simulink model "surgicalControl"  (R2016b)
settings: Solver=FixedStepAuto  StartTime=0.0  StopTime=100.0  RelTol=1e-3
libraries: simulink x3
settings Model: Creator=daniel  LastModifiedBy=migf1

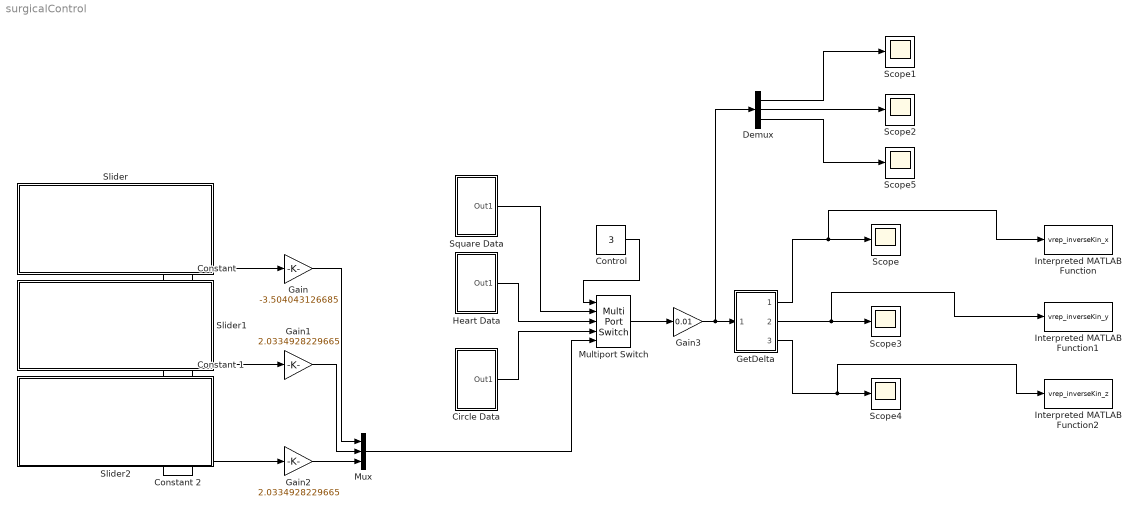
== system surgicalControl ==
  " GetDelta " : Subsystem
  " Constant " : Constant
  " Constant 1" : Constant
  " Constant 2" : Constant
  "Circle Data " : Subsystem
  "Control " : Constant  Value=3
  Demux : Demux  Outputs=3
  Gain : Gain  Gain=-3.504043126685
  Gain1 : Gain  Gain=2.0334928229665
  Gain2 : Gain  Gain=2.0334928229665
  Gain3 : Gain  Gain=0.01
  "Heart Data " : Subsystem
  Interpreted MATLAB Function : MATLABFcn  MATLABFcn=vrep_inverseKin_x
  Interpreted MATLAB Function1 : MATLABFcn  MATLABFcn=vrep_inverseKin_y
  Interpreted MATLAB Function2 : MATLABFcn  MATLABFcn=vrep_inverseKin_z
  Multiport Switch : MultiPortSwitch  Inputs=4
  Mux : Mux  Inputs=3
  Scope{,1..5} (6 alike) : Scope
  Slider : Subsystem  DialogController=hmiCreateDDGDialog  IsWebBlock=on  mask(MWDashboardBlock){webBlockId=4f94596f-dd6d-4e5e-bddc-7a8d913927f9, webBlockType=slider, ShowInLibBrowser=on, ShowInitialText=on, HMISrcModelName=surgicalControl}
      mask prompts: webBlockId "WebBlock Id"; webBlockType "WebBlock Type"; HMISrcModelName "Source Model"
      mask help: SimulinkHMI:dialogs:SliderDialogDesc
      mask Help: helpview([docroot '/mapfiles/simulink.map'], 'hmi_slider')
      mask Display:
      | if strcmp(get_param(bdroot(gcb),'BlockDiagramType'), 'library')
      |     image([(matlabroot) '/toolbox/simulink/hmi/icons/Slider.png']);
      | end
  Slider1 : Subsystem  DialogController=hmiCreateDDGDialog  IsWebBlock=on  mask(MWDashboardBlock){webBlockId=8aa996ad-7cd4-40fc-9a04-6a85939aea5d, webBlockType=slider, ShowInLibBrowser=on, ShowInitialText=on, HMISrcModelName=surgicalControl}
      mask prompts: webBlockId "WebBlock Id"; webBlockType "WebBlock Type"; HMISrcModelName "Source Model"
      mask help: SimulinkHMI:dialogs:SliderDialogDesc
      mask Help: helpview([docroot '/mapfiles/simulink.map'], 'hmi_slider')
      mask Display:
      | if strcmp(get_param(bdroot(gcb),'BlockDiagramType'), 'library')
      |     image([(matlabroot) '/toolbox/simulink/hmi/icons/Slider.png']);
      | end
  Slider2 : Subsystem  DialogController=hmiCreateDDGDialog  IsWebBlock=on  mask(MWDashboardBlock){webBlockId=1ddf6fd9-0225-4881-82ca-a25e179e2ab9, webBlockType=slider, ShowInLibBrowser=on, ShowInitialText=on, HMISrcModelName=surgicalControl}
      mask prompts: webBlockId "WebBlock Id"; webBlockType "WebBlock Type"; HMISrcModelName "Source Model"
      mask help: SimulinkHMI:dialogs:SliderDialogDesc
      mask Help: helpview([docroot '/mapfiles/simulink.map'], 'hmi_slider')
      mask Display:
      | if strcmp(get_param(bdroot(gcb),'BlockDiagramType'), 'library')
      |     image([(matlabroot) '/toolbox/simulink/hmi/icons/Slider.png']);
      | end
  "Square Data " : Subsystem
  wires:
  " GetDelta "/1(Out1) -> Interpreted MATLAB Function/1, Scope/1
  " GetDelta "/2(Out2) -> Interpreted MATLAB Function1/1, Scope3/1
  " GetDelta "/3(Out3) -> Interpreted MATLAB Function2/1, Scope4/1
  Multiport Switch/1 -> Gain3/1
  "Square Data "/1(Out1) -> Multiport Switch/2
  "Control "/1 -> Multiport Switch/1
  " Constant "/1 -> Gain/1
  " Constant 1"/1 -> Gain1/1
  " Constant 2"/1 -> Gain2/1
  Gain/1 -> Mux/1
  Gain1/1 -> Mux/2
  Gain2/1 -> Mux/3
  Mux/1 -> Multiport Switch/5
  "Heart Data "/1(Out1) -> Multiport Switch/3
  "Circle Data "/1(Out1) -> Multiport Switch/4
  Gain3/1 -> Demux/1, " GetDelta "/1(In1)
  Demux/2 -> Scope2/1
  Demux/1 -> Scope1/1
  Demux/3 -> Scope5/1

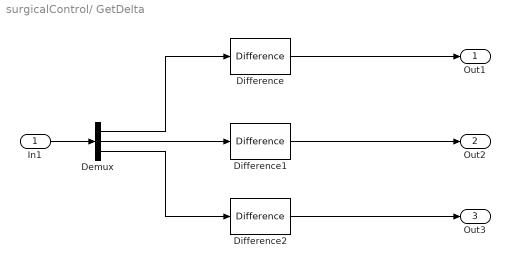
== system surgicalControl/ GetDelta  ==
  In1 : Inport
  Demux : Demux  Outputs=3
  Difference : simulink/Discrete/Difference  ICPrevInput=0  OutMin=[]  OutMax=[]  OutDataType=fixdt(1, 16)  OutScaling=2^-10  DoSatur=off
  Difference1 : simulink/Discrete/Difference  ICPrevInput=0  OutMin=[]  OutMax=[]  OutDataType=fixdt(1, 16)  OutScaling=2^-10  DoSatur=off
  Difference2 : simulink/Discrete/Difference  ICPrevInput=0  OutMin=[]  OutMax=[]  OutDataType=fixdt(1, 16)  OutScaling=2^-10  DoSatur=off
  Out1 : Outport
  Out2 : Outport  Port=2
  Out3 : Outport  Port=3
  wires:
  Difference1/1 -> Out2/1
  Difference/1 -> Out1/1
  Difference2/1 -> Out3/1
  In1/1 -> Demux/1
  Demux/1 -> Difference/1
  Demux/2 -> Difference1/1
  Demux/3 -> Difference2/1

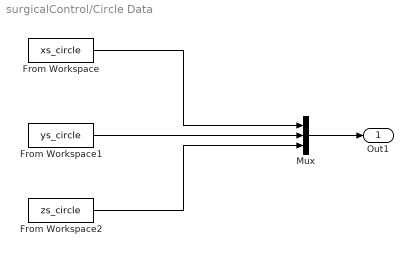
== system surgicalControl/Circle Data  ==
  From Workspace : FromWorkspace  VariableName=xs_circle  SampleTime=1
  From Workspace1 : FromWorkspace  VariableName=ys_circle  SampleTime=1
  From Workspace2 : FromWorkspace  VariableName=zs_circle  SampleTime=1
  Mux : Mux  Inputs=3
  Out1 : Outport
  wires:
  From Workspace/1 -> Mux/1
  From Workspace2/1 -> Mux/3
  Mux/1 -> Out1/1
  From Workspace1/1 -> Mux/2

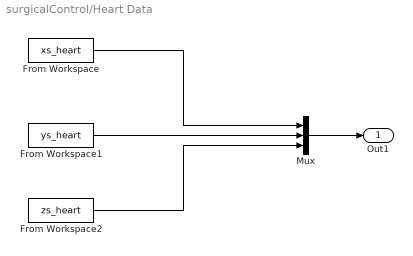
== system surgicalControl/Heart Data  ==
  From Workspace : FromWorkspace  VariableName=xs_heart  SampleTime=1
  From Workspace1 : FromWorkspace  VariableName=ys_heart  SampleTime=1
  From Workspace2 : FromWorkspace  VariableName=zs_heart  SampleTime=1
  Mux : Mux  Inputs=3
  Out1 : Outport
  wires:
  From Workspace/1 -> Mux/1
  From Workspace2/1 -> Mux/3
  Mux/1 -> Out1/1
  From Workspace1/1 -> Mux/2

== system surgicalControl/Slider ==

== system surgicalControl/Slider1 ==

== system surgicalControl/Slider2 ==

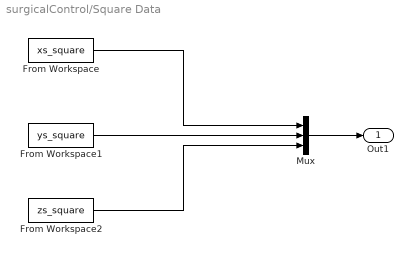
== system surgicalControl/Square Data  ==
  From Workspace : FromWorkspace  VariableName=xs_square  SampleTime=1
  From Workspace1 : FromWorkspace  VariableName=ys_square  SampleTime=1
  From Workspace2 : FromWorkspace  VariableName=zs_square  SampleTime=1
  Mux : Mux  Inputs=3
  Out1 : Outport
  wires:
  From Workspace/1 -> Mux/1
  From Workspace2/1 -> Mux/3
  Mux/1 -> Out1/1
  From Workspace1/1 -> Mux/2
